simulink model "VisionModel_v16_4"  (Simulink 7.6)
settings: Solver=FixedStepDiscrete  StartTime=0.0  StopTime=0  RelTol=1e-3
undefined symbols (not defined in the file or in its folder): Rec, SDTV
libraries: vipconversions x2
settings Model: Creator=Administrator  LastModifiedBy=root
settings OptimizationCC: OptimizeModelRefInitCode=on
settings RTWCC: SystemTargetFile=ert.tlc  GenCodeOnly=on  TemplateMakefile=ert_default_tmf  PostCodeGenCommand=packNGo(buildInfo, {'packType' 'flat'})  Description=Real-Time Workshop Embedded Coder  GenerateReport=on  ProcessScript=ert_make_rtw_hook  IncludeHyperlinkInReport=on  LaunchReport=on  TargetLang=C++
settings CodeAppCC: IgnoreCustomStorageClasses=off
settings ERTTargetCC: MultiwordLength=2048  GenerateSampleERTMain=on  IncludeMdlTerminateFcn=off  ERTCustomFileTemplate=example_file_process.tlc  ConvertIfToSwitch=off

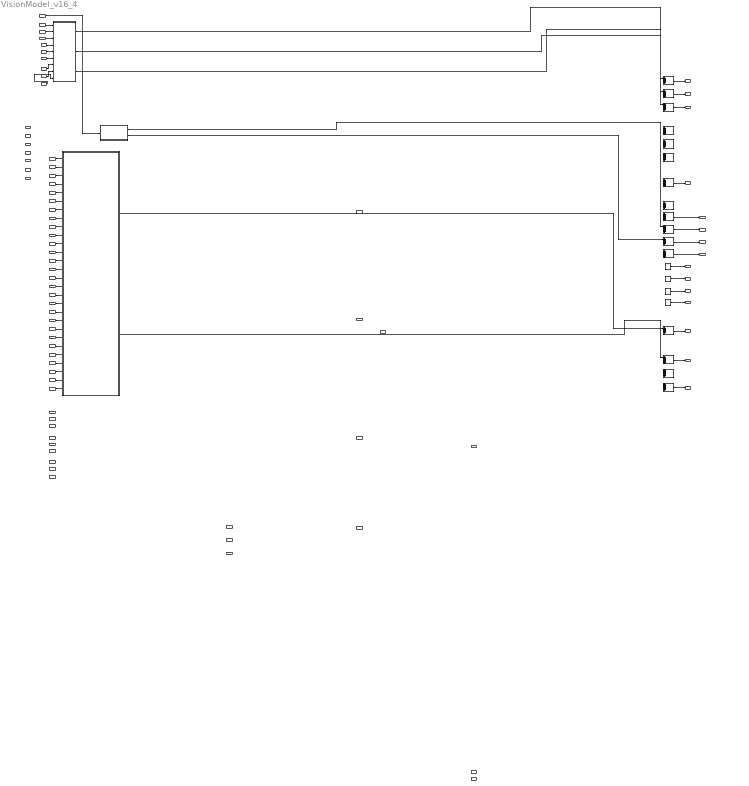
== system VisionModel_v16_4 ==
  note: Forward camera QImage array
  note: Down camera QImage array
  note: Forward
  note: Down
  note: Current target information
  note: Desired target information
  note: Mode and general target information
  note: Note: TargetFound, and the last three inputs to MotionController.mdl,
      | can be changed by the script, not the vision model.
  note: Path-following variables
      | DesiredPathDirection:
      | 0 = Use internal default
      | 1 = Take left path
      | 2 = Take right path
  R_forward_in : Inport  PortDimensions=Forward_Camera_Dimensions
  G_forward_in : Inport  Port=2  PortDimensions=Forward_Camera_Dimensions
  B_forward_in : Inport  Port=3  PortDimensions=Forward_Camera_Dimensions
  R_down_in : Inport  Port=4  PortDimensions=Down_Camera_Dimensions
  G_down_in : Inport  Port=5  PortDimensions=Down_Camera_Dimensions
  B_down_in : Inport  Port=6  PortDimensions=Down_Camera_Dimensions
  ModeSelect : Inport  Port=7
  OutputImage : Inport  Port=8
  DesiredPathDirection : Inport  Port=9
  DesiredBuoyColor : Inport  Port=10
  DesiredTorpedoColor : Inport  Port=11
  white_al : Inport  Port=12
  white_au : Inport  Port=13
  white_bl : Inport  Port=14
  white_bu : Inport  Port=15
  black_al : Inport  Port=16
  black_au : Inport  Port=17
  black_bl : Inport  Port=18
  black_bu : Inport  Port=19
  blue_al : Inport  Port=20
  blue_au : Inport  Port=21
  blue_bl : Inport  Port=22
  blue_bu : Inport  Port=23
  red_al : Inport  Port=24
  red_au : Inport  Port=25
  red_bl : Inport  Port=26
  red_bu : Inport  Port=27
  orange_al : Inport  Port=28
  orange_au : Inport  Port=29
  orange_bl : Inport  Port=30
  orange_bu : Inport  Port=31
  yellow_al : Inport  Port=32
  yellow_au : Inport  Port=33
  yellow_bl : Inport  Port=34
  yellow_bu : Inport  Port=35
  green_al : Inport  Port=36
  green_au : Inport  Port=37
  green_bl : Inport  Port=38
  green_bu : Inport  Port=39
  black_override : Inport  Port=40
  white_override : Inport  Port=41
  blue_override : Inport  Port=42
  red_override : Inport  Port=43
  orange_override : Inport  Port=44
  yellow_override : Inport  Port=45
  green_override : Inport  Port=46
  Scale_Forward_R : Inport  Port=47
  Scale_Forward_G : Inport  Port=48
  Scale_Forward_B : Inport  Port=49
  Scale_Forward_H : Inport  Port=50
  Scale_Forward_S : Inport  Port=51
  Scale_Forward_V : Inport  Port=52
  Scale_Down_R : Inport  Port=53
  Scale_Down_G : Inport  Port=54
  Scale_Down_B : Inport  Port=55
  Scale_Down_H : Inport  Port=56
  Scale_Down_S : Inport  Port=57
  Scale_Down_V : Inport  Port=58
  DeadReckonHeading : Inport  Port=59
  Add{,2..6,18..27} (16 alike) : Sum  Inputs=++++++
  ColorSelect : Subsystem  TreatAsAtomicUnit=on
  Constant{,1..3} (4 alike) : Constant  Value=0
  Forward Filter : Subsystem
  make_color_range : Stateflow chart  TreatAsAtomicUnit=on
  R_forward_out : Outport  OutDataTypeStr=double
  G_forward_out : Outport  Port=2  OutDataTypeStr=double
  B_forward_out : Outport  Port=3  OutDataTypeStr=double
  R_down_out : Outport  Port=4  OutDataTypeStr=double
  G_down_out : Outport  Port=5  OutDataTypeStr=double
  B_down_out : Outport  Port=6  OutDataTypeStr=double
  TargetSelect : Outport  Port=7  OutDataTypeStr=double
  TargetX : Outport  Port=8  OutDataTypeStr=double
  TargetY : Outport  Port=9  OutDataTypeStr=double
  TargetZ : Outport  Port=10  OutDataTypeStr=double
  TargetYaw : Outport  Port=11  OutDataTypeStr=double
  DesiredTargetX : Outport  Port=12  OutDataTypeStr=double
  DesiredTargetY : Outport  Port=13  OutDataTypeStr=double
  DesiredTargetZ : Outport  Port=14  OutDataTypeStr=double
  DesiredTargetYaw : Outport  Port=15  OutDataTypeStr=double
  TargetDetected : Outport  Port=16  OutDataTypeStr=double
  PathState : Outport  Port=17  OutDataTypeStr=double
  BuoyColors : Outport  Port=18  OutDataTypeStr=double
  FireAuthorization : Outport  Port=19  OutDataTypeStr=double
  TargetType : Outport  Port=20  OutDataTypeStr=double
  TargetSize : Outport  Port=21  OutDataTypeStr=double
  wires:
  R_forward_in/1 -> Forward Filter/1(R_in)
  G_forward_in/1 -> Forward Filter/2(G_in)
  B_forward_in/1 -> Forward Filter/3(B_in)
  Add3/1 -> TargetX/1
  Add4/1 -> TargetY/1
  Add5/1 -> TargetZ/1
  Add6/1 -> TargetYaw/1
  Add19/1 -> PathState/1
  Constant/1 -> DesiredTargetX/1
  Constant3/1 -> DesiredTargetYaw/1
  Constant2/1 -> DesiredTargetZ/1
  Constant1/1 -> DesiredTargetY/1
  Add21/1 -> FireAuthorization/1
  ModeSelect/1 -> ColorSelect/1(ModeSelect)
  Add/1 -> TargetSelect/1
  Add18/1 -> TargetDetected/1
  white_al/1 -> make_color_range/1(white_al)
  white_au/1 -> make_color_range/2(white_au)
  white_bl/1 -> make_color_range/3(white_bl)
  white_bu/1 -> make_color_range/4(white_bu)
  black_al/1 -> make_color_range/5(black_al)
  black_au/1 -> make_color_range/6(black_au)
  black_bl/1 -> make_color_range/7(black_bl)
  black_bu/1 -> make_color_range/8(black_bu)
  blue_al/1 -> make_color_range/9(blue_al)
  blue_au/1 -> make_color_range/10(blue_au)
  blue_bl/1 -> make_color_range/11(blue_bl)
  blue_bu/1 -> make_color_range/12(blue_bu)
  red_al/1 -> make_color_range/13(red_al)
  red_au/1 -> make_color_range/14(red_au)
  red_bl/1 -> make_color_range/15(red_bl)
  red_bu/1 -> make_color_range/16(red_bu)
  orange_al/1 -> make_color_range/17(orange_al)
  orange_au/1 -> make_color_range/18(orange_au)
  orange_bl/1 -> make_color_range/19(orange_bl)
  orange_bu/1 -> make_color_range/20(orange_bu)
  yellow_al/1 -> make_color_range/21(yellow_al)
  yellow_au/1 -> make_color_range/22(yellow_au)
  yellow_bl/1 -> make_color_range/23(yellow_bl)
  yellow_bu/1 -> make_color_range/24(yellow_bu)
  green_al/1 -> make_color_range/25(green_al)
  green_au/1 -> make_color_range/26(green_au)
  green_bl/1 -> make_color_range/27(green_bl)
  green_bu/1 -> make_color_range/28(green_bu)
  Add22/1 -> R_forward_out/1
  Add23/1 -> G_forward_out/1
  Add24/1 -> B_forward_out/1
  Scale_Forward_R/1 -> Forward Filter/4(Scale_Forward_R)
  Scale_Forward_G/1 -> Forward Filter/5(Scale_Forward_G)
  Scale_Forward_B/1 -> Forward Filter/6(Scale_Forward_B)
  Scale_Forward_H/1 -> Forward Filter/7(Scale_Forward_H)
  Scale_Forward_S/1 -> Forward Filter/8(Scale_Forward_S)
  Scale_Forward_V/1 -> Forward Filter/9(Scale_Forward_V)
  Forward Filter/1(R_out) -> Add22/1
  Forward Filter/2(G_out) -> Add23/1
  Forward Filter/3(B_out) -> Add24/1
  ColorSelect/1(ColorFilter) -> Add4/1
  ColorSelect/2(OutputSegmentedImage) -> Add5/1
  make_color_range/1(a_range) -> Add18/1
  make_color_range/2(b_range) -> Add19/1

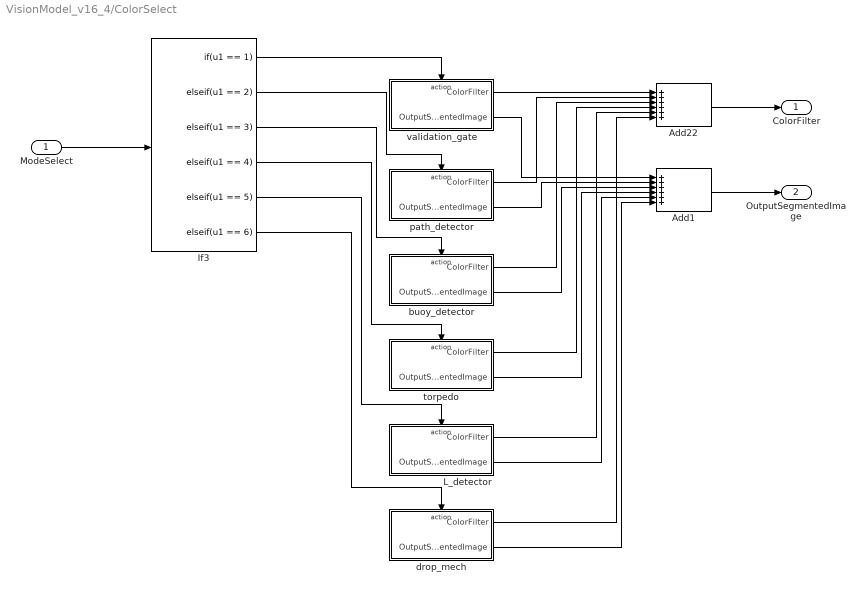
== system VisionModel_v16_4/ColorSelect ==
  ModeSelect : Inport
  Add1 : Sum  Inputs=++++++
  Add22 : Sum  Inputs=++++++
  If3 : If  IfExpression=u1 == 1  ElseIfExpressions=u1 == 2, u1 == 3, u1 == 4, u1 == 5, u1 == 6  ShowElse=off
  L_detector : Subsystem  TreatAsAtomicUnit=on
  buoy_detector : Subsystem  TreatAsAtomicUnit=on
  drop_mech : Subsystem  TreatAsAtomicUnit=on
  path_detector : Subsystem  TreatAsAtomicUnit=on
  torpedo : Subsystem  TreatAsAtomicUnit=on
  validation_gate : Subsystem  TreatAsAtomicUnit=on
  ColorFilter : Outport  OutDataTypeStr=double
  OutputSegmentedImage : Outport  Port=2  OutDataTypeStr=double
  wires:
  ModeSelect/1 -> If3/1
  If3/1 -> validation_gate/Action
  Add22/1 -> ColorFilter/1
  If3/2 -> path_detector/Action
  If3/3 -> buoy_detector/Action
  If3/4 -> torpedo/Action
  If3/5 -> L_detector/Action
  If3/6 -> drop_mech/Action
  Add1/1 -> OutputSegmentedImage/1
  validation_gate/1(ColorFilter) -> Add22/1
  validation_gate/2(OutputSegmentedImage) -> Add1/1
  path_detector/1(ColorFilter) -> Add22/2
  path_detector/2(OutputSegmentedImage) -> Add1/2
  buoy_detector/1(ColorFilter) -> Add22/3
  buoy_detector/2(OutputSegmentedImage) -> Add1/3
  torpedo/1(ColorFilter) -> Add22/4
  torpedo/2(OutputSegmentedImage) -> Add1/4
  L_detector/1(ColorFilter) -> Add22/5
  L_detector/2(OutputSegmentedImage) -> Add1/5
  drop_mech/1(ColorFilter) -> Add22/6
  drop_mech/2(OutputSegmentedImage) -> Add1/6

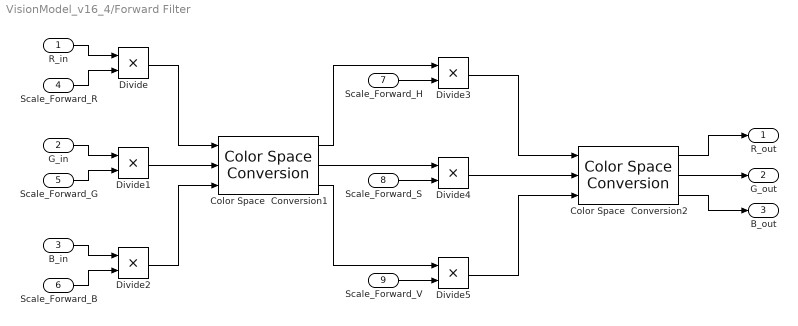
== system VisionModel_v16_4/Forward Filter ==
  R_in : Inport  PortDimensions=Forward_Camera_Dimensions
  G_in : Inport  Port=2  PortDimensions=Forward_Camera_Dimensions
  B_in : Inport  Port=3  PortDimensions=Forward_Camera_Dimensions
  Scale_Forward_R : Inport  Port=4
  Scale_Forward_G : Inport  Port=5
  Scale_Forward_B : Inport  Port=6
  Scale_Forward_H : Inport  Port=7
  Scale_Forward_S : Inport  Port=8
  Scale_Forward_V : Inport  Port=9
  Color Space  Conversion1 : vipconversions/Color Space  Conversion  conversion=Obsolete  conversionActive=R'G'B' to HSV  wp_str=D50  rec=Rec. 601 (SDTV)  sys=1125/60/2:1  imagePorts=Separate color signals
  Color Space  Conversion2 : vipconversions/Color Space  Conversion  conversion=Obsolete  conversionActive=HSV to R'G'B'  wp_str=D50  rec=Rec. 601 (SDTV)  sys=1125/60/2:1  imagePorts=Separate color signals
  Divide{,1..5} (6 alike) : Product  Inputs=**
  R_out : Outport  OutDataTypeStr=double
  G_out : Outport  Port=2  OutDataTypeStr=double
  B_out : Outport  Port=3  OutDataTypeStr=double
  wires:
  Color Space  Conversion2/1 -> R_out/1
  Color Space  Conversion2/2 -> G_out/1
  Color Space  Conversion2/3 -> B_out/1
  R_in/1 -> Divide/1
  Scale_Forward_R/1 -> Divide/2
  G_in/1 -> Divide1/1
  Scale_Forward_G/1 -> Divide1/2
  B_in/1 -> Divide2/1
  Scale_Forward_B/1 -> Divide2/2
  Divide/1 -> Color Space  Conversion1/1
  Divide1/1 -> Color Space  Conversion1/2
  Divide2/1 -> Color Space  Conversion1/3
  Scale_Forward_H/1 -> Divide3/2
  Scale_Forward_S/1 -> Divide4/2
  Scale_Forward_V/1 -> Divide5/2
  Color Space  Conversion1/1 -> Divide3/1
  Color Space  Conversion1/2 -> Divide4/1
  Color Space  Conversion1/3 -> Divide5/1
  Divide4/1 -> Color Space  Conversion2/2
  Divide3/1 -> Color Space  Conversion2/1
  Divide5/1 -> Color Space  Conversion2/3

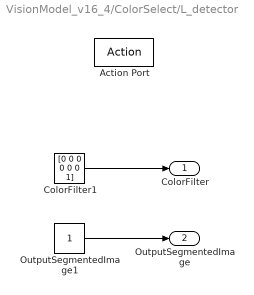
== system VisionModel_v16_4/ColorSelect/L_detector ==
  Action Port : ActionPort  ActionType=elseif
  ColorFilter1 : Constant  Value=[0 0 0 0 0 0 1]  SampleTime=-1
  OutputSegmentedImage1 : Constant  SampleTime=-1
  ColorFilter : Outport  OutDataTypeStr=double
  OutputSegmentedImage : Outport  Port=2  OutDataTypeStr=double
  wires:
  ColorFilter1/1 -> ColorFilter/1
  OutputSegmentedImage1/1 -> OutputSegmentedImage/1

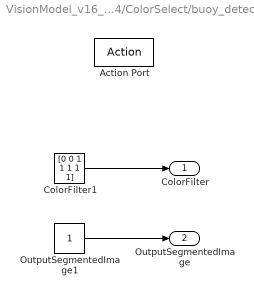
== system VisionModel_v16_4/ColorSelect/buoy_detector ==
  Action Port : ActionPort  ActionType=elseif
  ColorFilter1 : Constant  Value=[0 0 1 1 1 1 1]  SampleTime=-1
  OutputSegmentedImage1 : Constant  SampleTime=-1
  ColorFilter : Outport  OutDataTypeStr=double
  OutputSegmentedImage : Outport  Port=2  OutDataTypeStr=double
  wires:
  ColorFilter1/1 -> ColorFilter/1
  OutputSegmentedImage1/1 -> OutputSegmentedImage/1

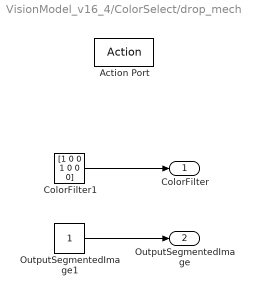
== system VisionModel_v16_4/ColorSelect/drop_mech ==
  Action Port : ActionPort  ActionType=elseif
  ColorFilter1 : Constant  Value=[1 0 0 1 0 0 0]  SampleTime=-1
  OutputSegmentedImage1 : Constant  SampleTime=-1
  ColorFilter : Outport  OutDataTypeStr=double
  OutputSegmentedImage : Outport  Port=2  OutDataTypeStr=double
  wires:
  OutputSegmentedImage1/1 -> OutputSegmentedImage/1
  ColorFilter1/1 -> ColorFilter/1

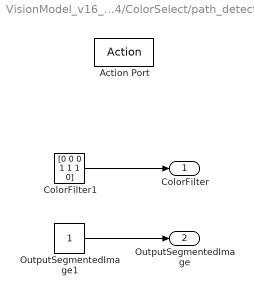
== system VisionModel_v16_4/ColorSelect/path_detector ==
  Action Port : ActionPort  ActionType=elseif
  ColorFilter1 : Constant  Value=[0 0 0 1 1 1 0]  SampleTime=-1
  OutputSegmentedImage1 : Constant  SampleTime=-1
  ColorFilter : Outport  OutDataTypeStr=double
  OutputSegmentedImage : Outport  Port=2  OutDataTypeStr=double
  wires:
  OutputSegmentedImage1/1 -> OutputSegmentedImage/1
  ColorFilter1/1 -> ColorFilter/1

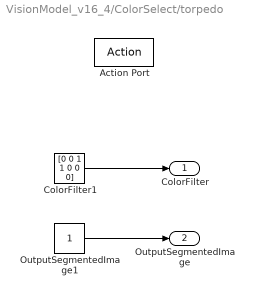
== system VisionModel_v16_4/ColorSelect/torpedo ==
  Action Port : ActionPort  ActionType=elseif
  ColorFilter1 : Constant  Value=[0 0 1 1 0 0 0]  SampleTime=-1
  OutputSegmentedImage1 : Constant  SampleTime=-1
  ColorFilter : Outport  OutDataTypeStr=double
  OutputSegmentedImage : Outport  Port=2  OutDataTypeStr=double
  wires:
  OutputSegmentedImage1/1 -> OutputSegmentedImage/1
  ColorFilter1/1 -> ColorFilter/1

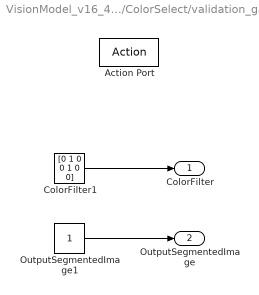
== system VisionModel_v16_4/ColorSelect/validation_gate ==
  Action Port : ActionPort  ActionType=then
  ColorFilter1 : Constant  Value=[0 1 0 0 1 0 0]  SampleTime=-1
  OutputSegmentedImage1 : Constant  SampleTime=-1
  ColorFilter : Outport  OutDataTypeStr=double
  OutputSegmentedImage : Outport  Port=2  OutDataTypeStr=double
  wires:
  ColorFilter1/1 -> ColorFilter/1
  OutputSegmentedImage1/1 -> OutputSegmentedImage/1

== matlab function make_color_range ==
  data: a_range output double; b_range output double; white_al input double; white_au input double; white_bl input double; white_bu input double; black_al input double; black_au input double; black_bl input double; black_bu input double; blue_al input double; blue_au input double; blue_bl input double; blue_bu input double; red_al input double; red_au input double; red_bl input double; red_bu input double; orange_al input double; orange_au input double; orange_bl input double; orange_bu input double; yellow_al input double; yellow_au input double; yellow_bl input double; yellow_bu input double; green_al input double; green_au input double; green_bl input double; green_bu input double
function [a_range, b_range] = make_color_range(white_al, white_au, white_bl, white_bu, black_al, black_au, black_bl, black_bu, blue_al, blue_au, blue_bl, blue_bu, red_al, red_au, red_bl, red_bu, orange_al, orange_au, orange_bl, orange_bu, yellow_al, yellow_au, yellow_bl, yellow_bu, green_al, green_au, green_bl, green_bu)

% This function forms two compact matrices which pass all color range
%   information to other functions in the model


% Initialize
a_range = zeros(2, 7);
b_range = zeros(2, 7);


% Assign values to color range matrices
a_range(1, 1) = white_al;
a_range(2, 1) = white_au;
b_range(1, 1) = white_bl;
b_range(2, 1) = white_bu;

a_range(1, 2) = black_al;
a_range(2, 2) = black_au;
b_range(1, 2) = black_bl;
b_range(2, 2) = black_bu;

a_range(1, 3) = blue_al;
a_range(2, 3) = blue_au;
b_range(1, 3) = blue_bl;
b_range(2, 3) = blue_bu;

a_range(1, 4) = red_al;
a_range(2, 4) = red_au;
b_range(1, 4) = red_bl;
b_range(2, 4) = red_bu;

a_range(1, 5) = orange_al;
a_range(2, 5) = orange_au;
b_range(1, 5) = orange_bl;
b_range(2, 5) = orange_bu;

a_range(1, 6) = yellow_al;
a_range(2, 6) = yellow_au;
b_range(1, 6) = yellow_bl;
b_range(2, 6) = yellow_bu;

a_range(1, 7) = green_al;
a_range(2, 7) = green_au;
b_range(1, 7) = green_bl;
b_range(2, 7) = green_bu;


return
